simulink model "separator"  (R2018b)
settings: Solver=VariableStepAuto  StartTime=0.0  StopTime=100  RelTol=1e-3
settings Model: Creator=gv281  LastModifiedBy=jh2044

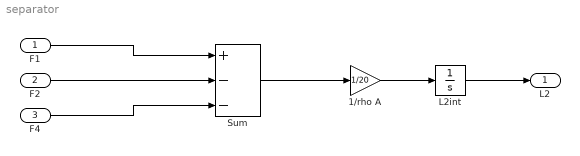
== system separator ==
  F1 : Inport
  "F2 " : Inport  Port=2
  F4 : Inport  Port=3
  1/rho A : Gain  Gain=1/20
  L2int : Integrator
  Sum : Sum  Inputs=+--
  L2 : Outport
  wires:
  1/rho A/1 -> L2int/1
  Sum/1 -> 1/rho A/1
  F4/1 -> Sum/3
  "F2 "/1 -> Sum/2
  F1/1 -> Sum/1
  L2int/1 -> L2/1
